simulink model "curentulrotoric"  (R2023b)
settings: Solver=VariableStepAuto  StartTime=0.0  StopTime=10.0  RelTol=1e-3
values from neighbouring files (symbols this model uses):
  k = 0.035    [untitled2.m]
settings Model: Creator=diana.forrai  LastModifiedBy=diana.forrai

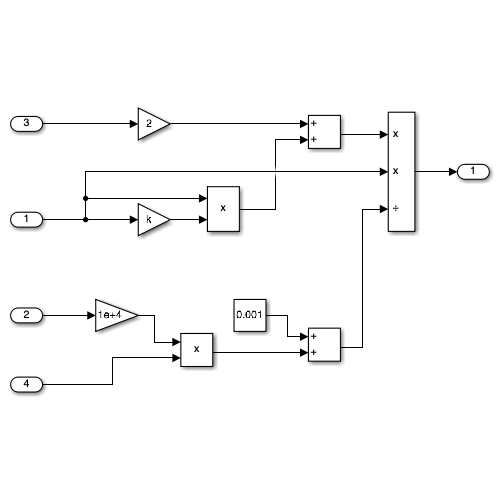
[thumbnail: Simulink's stored preview of the top-level diagram]
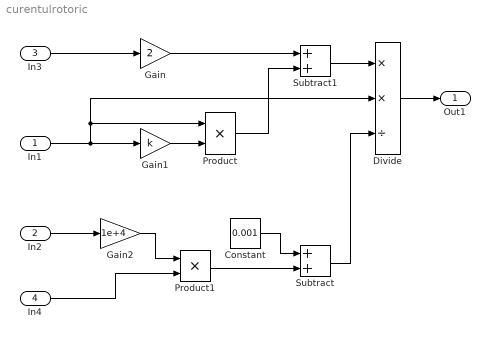
== system curentulrotoric ==
  In1 : Inport
  In2 : Inport  Port=2
  In3 : Inport  Port=3
  In4 : Inport  Port=4
  Constant : Constant  Value=0.001
  Divide : Product  Inputs=**/
  Gain : Gain  Gain=2
  Gain1 : Gain  Gain=k
  Gain2 : Gain  Gain=1e+4
  Product : Product
  Product1 : Product
  Subtract : Sum
  Subtract1 : Sum
  Out1 : Outport
  wires:
  In1/1 -> Divide/2, Product/1, Gain1/1
  Gain1/1 -> Product/2
  Product/1 -> Subtract1/2
  Gain/1 -> Subtract1/1
  In3/1 -> Gain/1
  In2/1 -> Gain2/1
  Gain2/1 -> Product1/1
  In4/1 -> Product1/2
  Constant/1 -> Subtract/1
  Product1/1 -> Subtract/2
  Subtract1/1 -> Divide/1
  Subtract/1 -> Divide/3
  Divide/1 -> Out1/1
